simulink model "predictive_pid"  (Simulink 5.0)
settings: Solver=ode45  StartTime=0.0  StopTime=350.0  RelTol=1e-3
settings Model: LastModifiedBy=pari

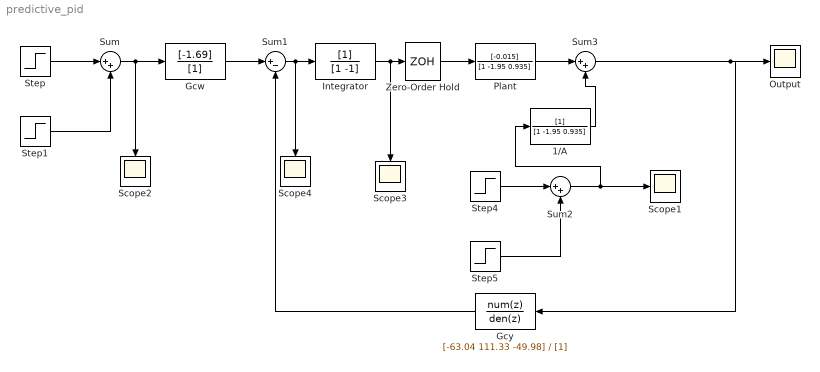
== system predictive_pid ==
  1/A : DiscreteFilter  Denominator=[1 -1.95 0.935]
  Gcw : DiscreteFilter  Numerator=[-1.69]  Denominator=[1]
  Gcy : DiscreteFilter  Orientation=left  Numerator=[-63.04 111.33 -49.98]  Denominator=[1]
  Integrator : DiscreteFilter  Denominator=[1 -1]
  Output : Scope
      settings: YMin=-0.5  YMax=2
  Plant : DiscreteFilter  Numerator=[-0.015]  Denominator=[1 -1.95 0.935]
  Scope{1..4} (4 alike) : Scope
      Scope2 settings: Orientation=down  SaveName=ScopeData2
      Scope3 settings: Orientation=down  SaveName=ScopeData3
      Scope4 settings: Orientation=down  SaveName=ScopeData4
  Step : Step  Time=50  SampleTime=1
  Step1 : Step  Time=200  After=-1  SampleTime=1
  Step4 : Step  Time=100  After=0.1  SampleTime=1
  Step5 : Step  Time=150  After=-0.1  SampleTime=1
  Sum : Sum  Inputs=|++  SaturateOnIntegerOverflow=on
  Sum1 : Sum  Inputs=|+-  SaturateOnIntegerOverflow=on
  Sum2 : Sum  Inputs=|++  SaturateOnIntegerOverflow=on
  Sum3 : Sum  Inputs=|++  SaturateOnIntegerOverflow=on
  Zero-Order Hold : ZeroOrderHold
  wires:
  Step1/1 -> Sum/2
  Step/1 -> Sum/1
  Sum/1 -> Gcw/1, Scope2/1
  Gcw/1 -> Sum1/1
  Step5/1 -> Sum2/2
  Sum2/1 -> Scope1/1, 1/A/1
  Plant/1 -> Sum3/1
  Sum3/1 -> Output/1, Gcy/1
  Step4/1 -> Sum2/1
  Gcy/1 -> Sum1/2
  Sum1/1 -> Integrator/1, Scope4/1
  Integrator/1 -> Scope3/1, Zero-Order Hold/1
  Zero-Order Hold/1 -> Plant/1
  1/A/1 -> Sum3/2
